simulink model "VSI_LL_IC_"  (R2018a)
settings: Solver=ode23t  StartTime=0  StopTime=0.5  MaxStep=.1e-6  RelTol=1e-4  AbsTol=1e-5  EnableMultiTasking=on
InitFcn:
  | VSI_AFE_parameters_G1_s
values from neighbouring files (symbols this model uses):
  DeadTime = 0.0e-6    (= 0)    [VSI_AFE_parameters_G1_s.m]
  f = 400    [VSI_AFE_parameters_G1_s.m]
  Idref_VSI = 1*11.03    (= 11.03)    [VSI_AFE_parameters_G1_s.m]
  Iqref_VSI = -0    (= 0)    [VSI_AFE_parameters_G1_s.m]
  Ki_PLL_AFE = 1    [VSI_AFE_parameters_G1_s.m]
  Ki_PLL_VSI = 3964    [VSI_AFE_parameters_G1_s.m]
  Kii_AFE = 46.5421*270    (= 12566.367)    [VSI_AFE_parameters_G1_s.m]
  Kii_VSI = 10*628.3185/Vdc    (= 23.2710555556)    [VSI_AFE_parameters_G1_s.m]
  Kipq_VSI = 70    [VSI_AFE_parameters_G1_s.m]
  Kp_PLL_AFE = 0.2    [VSI_AFE_parameters_G1_s.m]
  Kp_PLL_VSI = 8.921    [VSI_AFE_parameters_G1_s.m]
  Kpi_AFE = 0.0116*270    (= 3.132)    [VSI_AFE_parameters_G1_s.m]
  Kpi_VSI = 6.2832/Vdc    (= 0.0232711111111)    [VSI_AFE_parameters_G1_s.m]
  Kppq_VSI = 70*4e-5    (= 0.0028)    [VSI_AFE_parameters_G1_s.m]
  Kpv_AFE = 0.0462    [VSI_AFE_parameters_G1_s.m]
  La = 1000e-6    (= 0.001)    [VSI_AFE_parameters_G1_s.m]
  Lb = 1000e-6    (= 0.001)    [VSI_AFE_parameters_G1_s.m]
  Lc = 1000e-6    (= 0.001)    [VSI_AFE_parameters_G1_s.m]
  PWM_Cycle = 4000    [VSI_AFE_parameters_G1_s.m]
  RLa = 0.100    (= 0.1)    [VSI_AFE_parameters_G1_s.m]
  RLb = 0.100    (= 0.1)    [VSI_AFE_parameters_G1_s.m]
  RLc = 0.100    (= 0.1)    [VSI_AFE_parameters_G1_s.m]
  Vdc = 270/1    (= 270)    [VSI_AFE_parameters_G1_s.m]
  Vfd = 0.75    [VSI_AFE_parameters_G1_s.m]
  Vfs = 1.0    (= 1)    [VSI_AFE_parameters_G1_s.m]
  Vsm = Vse*sqrt(2)-8.2/sqrt(2)*Rss    [VSI_AFE_parameters_G1_s.m]
libraries: powerlib x24, cstblocks x10, simulink x2, powerlib_extras x1
settings Model: Creator=marko  LastModifiedBy=wenbo
settings SolverCC: AutoScaleAbsTol=off  MaxConsecutiveMinStep=10  ZeroCrossAlgorithm=Adaptive  AlgebraicLoopSolver=LineSearch
settings DataIOCC: SaveFinalState=on  SaveFormat=Array  SignalLoggingSaveFormat=ModelDataLogs
settings OptimizationCC: ExpressionDepthLimit=2147483647  LifeSpan=inf
settings DebuggingCC: UnderspecifiedInitializationDetection=Classic  MergeDetectMultiDrivingBlocksExec=none  IgnoredZcDiagnostic=none  SolverPrmCheckMsg=warning  FcnCallInpInsideContextMsg=warning  StateNameClashWarn=warning  SFUnexpectedBacktrackingDiag=warning  SFNoUnconditionalDefaultTransitionDiag=warning  SFExecutionAtInitializationDiag=none
settings HardwareCC: ProdBitPerPointer=32  ProdBitPerSizeT=32  ProdBitPerPtrDiffT=32  ProdLargestAtomicFloat=None  ProdIntDivRoundTo=Undefined  ProdEndianess=Unspecified  ProdWordSize=32  ProdHWDeviceType=32-bit Generic
settings ModelReferenceCC: PropagateSignalLabelsOutOfModel=off
settings CodeAppCC: StateflowObjectComments=on
settings GRTTargetCC: TargetLangStandard=C89/C90 (ANSI)  GeneratePreprocessorConditionals=Disable all  CombineOutputUpdateFcns=off  GRTInterface=on
settings ConfigComp: CovMetricSettings=dw  CovHtmlReporting=on  CovSaveCumulativeToWorkspaceVar=on  CovSaveSingleToWorkspaceVar=on  CovExternalEMLEnable=off
settings SimscapeCC: SimscapeNormalizeSystem=off

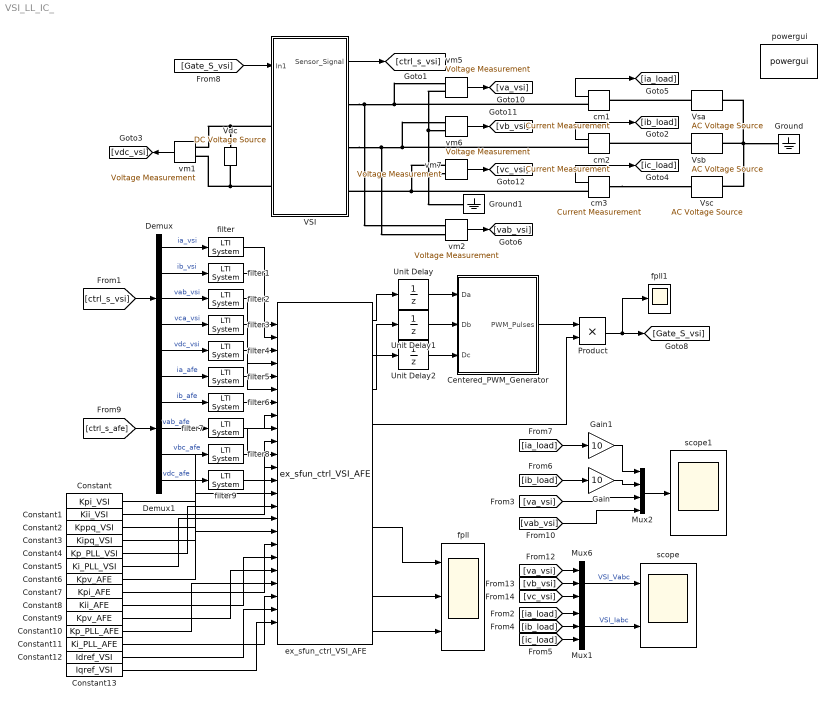
== system VSI_LL_IC_ ==
  Centered_PWM_Generator : Subsystem
  Constant : Constant  Value=Kpi_VSI
  Constant1 : Constant  Value=Kii_VSI
  Constant10 : Constant  Value=Kp_PLL_AFE
  Constant11 : Constant  Value=Ki_PLL_AFE
  Constant12 : Constant  Value=Idref_VSI
  Constant13 : Constant  Value=Iqref_VSI
  Constant2 : Constant  Value=Kppq_VSI
  Constant3 : Constant  Value=Kipq_VSI
  Constant4 : Constant  Value=Kp_PLL_VSI
  Constant5 : Constant  Value=Ki_PLL_VSI
  Constant6 : Constant  Value=Kpv_AFE
  Constant7 : Constant  Value=Kpi_AFE
  Constant8 : Constant  Value=Kii_AFE
  Constant9 : Constant  Value=Kpv_AFE
  Demux : Demux  Outputs=5
  Demux1 : Demux  Outputs=5
  Gain : Gain  Gain=10
  Gain1 : Gain  Gain=10
  Ground : powerlib/Elements/Ground  LConnTagsString=a
  Ground1 : powerlib/Elements/Ground  LConnTagsString=a
  Mux1 : Mux  Inputs=3
  Mux2 : Mux
  Mux6 : Mux  Inputs=3
  Product : Product  RndMeth=Zero
  Unit Delay : UnitDelay  SampleTime=-1
  Unit Delay1 : UnitDelay  SampleTime=-1
  Unit Delay2 : UnitDelay  SampleTime=-1
  VSI : Subsystem
  Vdc : powerlib/Electrical Sources/DC Voltage Source  Amplitude=Vdc  Measurements=None
  Vsa : powerlib/Electrical Sources/AC Voltage Source  Amplitude=Vsm  Phase=90  Frequency=f  SampleTime=0  Measurements=None  BusType=swing  Pref=10e3  Qref=0  Qmin=-inf  Qmax=+inf
  Vsb : powerlib/Electrical Sources/AC Voltage Source  Amplitude=Vsm  Phase=90-120  Frequency=f  SampleTime=0  Measurements=None  BusType=swing  Pref=10e3  Qref=0  Qmin=-inf  Qmax=+inf
  Vsc : powerlib/Electrical Sources/AC Voltage Source  Amplitude=Vsm  Phase=90+120  Frequency=f  SampleTime=0  Measurements=None  BusType=swing  Pref=10e3  Qref=0  Qmin=-inf  Qmax=+inf
  cm1 : powerlib/Measurements/Current Measurement  PhasorSimulation=off  OutputType=Complex  PSBequivalent=0
  cm2 : powerlib/Measurements/Current Measurement  PhasorSimulation=off  OutputType=Complex  PSBequivalent=0
  cm3 : powerlib/Measurements/Current Measurement  PhasorSimulation=off  OutputType=Complex  PSBequivalent=0
  ex_sfun_ctrl_VSI_AFE : S-Function  FunctionName=ex_sfun_ctrl_VSI_AFE  SFunctionDeploymentMode=off  EnableBusSupport=off  mask(Legacy Function){SFunctionSpec=void epwm1_isr(double y1[1], double y2[1], double y3[1], double y4[1], double y5[1], double y6[1], double y7[1], double y8[1], double y9[1], double u1, double u2, double u3, double u4, double u5, double u6, double u7, double u8, double u9, double u10), ShowSpec=off}
      mask prompts: ShowSpec "Display function specification"
      mask help:
      | This block allows you to call the legacy functions specified by the following Legacy Code Tool definition:
      | def.SFunctionName = 'ex_sfun_ctrl_VSI_AFE';
      | def.OutputFcnSpec = 'void epwm1_isr(double y1[1], double y2[1], double y3[1], double y4[1], double y5[1], double y6[1], double y7[1], double y8[1], double y9[1], double u1, double u2, double u3, double u4, double u5, double u6, double u7, double u8, double u9, double u10)';
      | def.HeaderFiles = {'math.h'};
      | def.SourceFiles = {'epwm1_isr.c'};
      | def.SampleTime = 5e-005;
      mask Help: <p>This block was generated automatically by the Legacy Code Tool. For detailed help on this tool, call<a href="matlab:legacy_code('help')"> legacy_code('help')</a>.</p>
      mask Callback ShowSpec:
      | if strcmp(get_param(gcbh, 'ShowSpec'), 'on')
      |   set_param(gcbh, 'MaskDisplay', sprintf('fprintf(''%s'');', get_param(gcbh, 'SFunctionSpec')));
      | else
      |   set_param(gcbh, 'MaskDisplay', sprintf('fprintf(''%s'');', get_param(gcbh, 'FunctionName')));
      | end
      mask Display: fprintf('ex_sfun_ctrl_VSI_AFE');
  filter{,1..9} (10 alike) : cstblocks/LTI System  sys=tf_filter  IC=[]
  fpll : Scope  NumInputPorts=3
  fpll1 : Scope
  powergui : powerlib/powergui  Priority=1  SimulationMode=Continuous  SampleTime=50e-6  frequency=60  Iterations=50  frequencyindice=0  Pbase=100e6  ErrMax=1e-4  UnitsV=kV  UnitsW=MW  buscounter=0  FunctionMessages=off  echomessages=off  EnableUseOfTLC=off  CurrentSourceSwitches=off  DisableSnubberDevices=off  DisableRonSwitches=off  DisableVfSwitches=off  DisplayEquations=off  SolverType=Tustin  Interpol=off  ExternalGateDelay=off  methode=off  Ts=0  x0status=blocks  SPID=on  SwTol=0  HookPort=off  RestoreLinks=warning  ResistiveCurrentMeasurement=off  Frange=[0:2:500]  Ylog=off  Xlog=on  ShowGrid=off  save=off  variable=ZData  structure=ia_L  ZoomFFT=on  StartTime=0.1  cycles=1  DisplayStyle=1  fundamental=400  FreqAxis=off  MaxFrequency=100000  frequencyindicesteady=400  RmsSteady=1  display=off
  scope : Scope  NumInputPorts=2
  scope1 : Scope
  vm{1..2,5..7} (5 alike) : powerlib/Measurements/Voltage Measurement  PhasorSimulation=off  OutputType=Complex  PSBequivalent=0
  wires:
  vm5/1 -> [va_vsi]
  vm6/1 -> [vb_vsi]
  vm7/1 -> [vc_vsi]
  [va_vsi] -> Mux6/1
  [vb_vsi] -> Mux6/2
  [vc_vsi] -> Mux6/3
  Mux6/1 -> scope/1  "VSI_Vabc"
  Unit Delay/1 -> Centered_PWM_Generator/1(Da)
  Unit Delay1/1 -> Centered_PWM_Generator/2(Db)
  Unit Delay2/1 -> Centered_PWM_Generator/3(Dc)
  Demux/1 -> filter/1  "ia_vsi"
  Demux/2 -> filter1/1  "ib_vsi"
  Demux/3 -> filter2/1  "vab_vsi"
  Demux/4 -> filter3/1  "vca_vsi"
  Demux/5 -> filter4/1  "vdc_vsi"
  VSI/1(Sensor_Signal) -> [ctrl_s_vsi]
  [ctrl_s_vsi] -> Demux/1
  [Gate_S_vsi] -> VSI/1(In1)
  Demux1/1 -> filter5/1  "ia_afe"
  Demux1/2 -> filter6/1  "ib_afe"
  Demux1/3 -> filter7/1  "vab_afe"
  Demux1/4 -> filter8/1  "vbc_afe"
  Demux1/5 -> filter9/1  "vdc_afe"
  [ctrl_s_afe] -> Demux1/1
  ex_sfun_ctrl_VSI_AFE/1 -> Unit Delay/1
  ex_sfun_ctrl_VSI_AFE/2 -> Unit Delay1/1
  ex_sfun_ctrl_VSI_AFE/3 -> Unit Delay2/1
  filter/1 -> ex_sfun_ctrl_VSI_AFE/1
  filter1/1 -> ex_sfun_ctrl_VSI_AFE/2
  filter2/1 -> ex_sfun_ctrl_VSI_AFE/3
  filter3/1 -> ex_sfun_ctrl_VSI_AFE/4
  filter4/1 -> ex_sfun_ctrl_VSI_AFE/5
  filter5/1 -> ex_sfun_ctrl_VSI_AFE/6
  filter6/1 -> ex_sfun_ctrl_VSI_AFE/7
  filter7/1 -> ex_sfun_ctrl_VSI_AFE/8
  filter8/1 -> ex_sfun_ctrl_VSI_AFE/9
  filter9/1 -> ex_sfun_ctrl_VSI_AFE/10
  vm1/1 -> [vdc_vsi]
  Mux1/1 -> scope/2  "VSI_Iabc"
  [ia_load] -> Mux1/1
  [ib_load] -> Mux1/2
  [ic_load] -> Mux1/3
  Product/1 -> [Gate_S_vsi], fpll1/1
  Centered_PWM_Generator/1(PWM_Pulses) -> Product/1
  ex_sfun_ctrl_VSI_AFE/4 -> Product/2
  Constant/1 -> ex_sfun_ctrl_VSI_AFE/11
  Constant1/1 -> ex_sfun_ctrl_VSI_AFE/12
  Constant2/1 -> ex_sfun_ctrl_VSI_AFE/13
  Constant3/1 -> ex_sfun_ctrl_VSI_AFE/14
  Constant4/1 -> ex_sfun_ctrl_VSI_AFE/15
  Constant5/1 -> ex_sfun_ctrl_VSI_AFE/16
  Constant6/1 -> ex_sfun_ctrl_VSI_AFE/17
  Constant7/1 -> ex_sfun_ctrl_VSI_AFE/18
  Constant8/1 -> ex_sfun_ctrl_VSI_AFE/19
  Constant9/1 -> ex_sfun_ctrl_VSI_AFE/20
  Constant10/1 -> ex_sfun_ctrl_VSI_AFE/21
  Constant11/1 -> ex_sfun_ctrl_VSI_AFE/22
  Constant12/1 -> ex_sfun_ctrl_VSI_AFE/23
  Constant13/1 -> ex_sfun_ctrl_VSI_AFE/24
  [ib_load] -> Gain/1
  Mux2/1 -> scope1/1
  ex_sfun_ctrl_VSI_AFE/9 -> fpll/2
  ex_sfun_ctrl_VSI_AFE/10 -> fpll/3
  ex_sfun_ctrl_VSI_AFE/7 -> fpll/1
  vm2/1 -> [vab_vsi]
  [ia_load] -> Gain1/1
  Gain1/1 -> Mux2/1
  Gain/1 -> Mux2/2
  [va_vsi] -> Mux2/3
  [vab_vsi] -> Mux2/4
  cm1/1 -> [ia_load]
  cm2/1 -> [ib_load]
  cm3/1 -> [ic_load]
  connections:
  VSI/LConn1 -- Vdc/RConn1 -- vm1/LConn1
  VSI/LConn2 -- Vdc/LConn1 -- vm1/LConn2
  vm7/LConn1 -- cm3/RConn1 -- VSI/RConn3
  VSI/RConn2 -- vm2/LConn2 -- vm6/LConn1 -- cm2/RConn1
  VSI/RConn1 -- vm2/LConn1 -- vm5/LConn1 -- cm1/RConn1
  Vsa/LConn1 -- Vsc/LConn1 -- Vsb/LConn1 -- Ground/LConn1
  vm5/LConn2 -- vm6/LConn2 -- Ground1/LConn1 -- vm7/LConn2
  cm3/LConn1 -- Vsc/RConn1
  Vsb/RConn1 -- cm2/LConn1
  Vsa/RConn1 -- cm1/LConn1

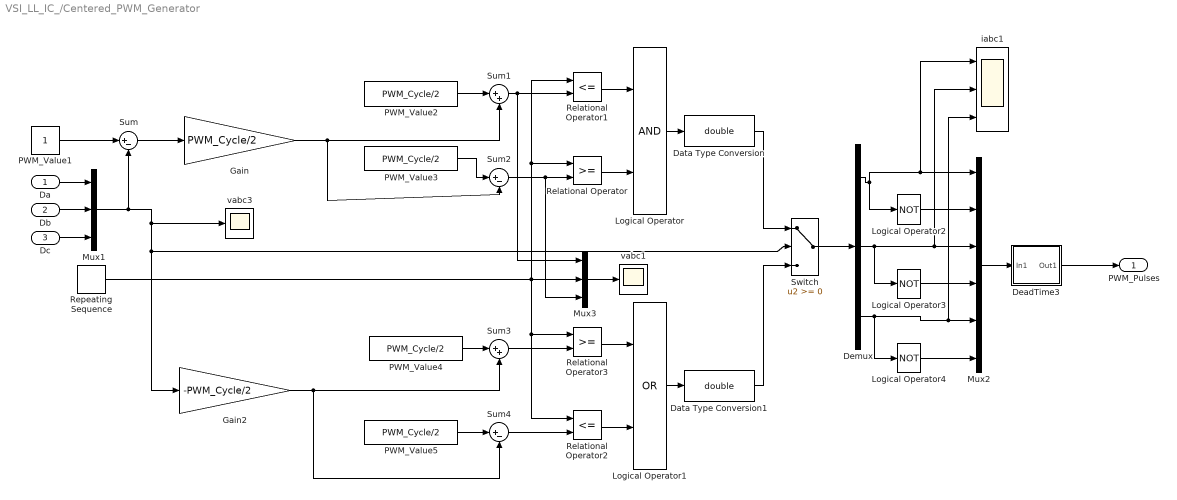
== system VSI_LL_IC_/Centered_PWM_Generator ==
  Da : Inport
  Db : Inport  Port=2
  Dc : Inport  Port=3
  Data Type Conversion : DataTypeConversion  OutDataTypeStr=double
  Data Type Conversion1 : DataTypeConversion  OutDataTypeStr=double
  DeadTime3 : Subsystem
  Demux : Demux  Outputs=3
  Gain : Gain  Gain=PWM_Cycle/2
  Gain2 : Gain  Gain=-PWM_Cycle/2
  Logical Operator : Logic  AllPortsSameDT=off  OutDataTypeStr=boolean
  Logical Operator1 : Logic  Operator=OR  AllPortsSameDT=off  OutDataTypeStr=boolean
  Logical Operator2 : Logic  Operator=NOT  OutDataTypeStr=float('double')
  Logical Operator3 : Logic  Operator=NOT  OutDataTypeStr=float('double')
  Logical Operator4 : Logic  Operator=NOT  OutDataTypeStr=float('double')
  Mux1 : Mux  Inputs=3
  Mux2 : Mux  Inputs=6
  Mux3 : Mux  Inputs=3
  PWM_Value1 : Constant
  PWM_Value{2..5} (4 alike) : Constant  Value=PWM_Cycle/2
  Relational Operator : RelationalOperator  OutDataTypeStr=boolean  RndMeth=Nearest
  Relational Operator1 : RelationalOperator  Operator=<=  OutDataTypeStr=boolean  RndMeth=Nearest
  Relational Operator2 : RelationalOperator  Operator=<=  OutDataTypeStr=boolean  RndMeth=Nearest
  Relational Operator3 : RelationalOperator  OutDataTypeStr=boolean  RndMeth=Nearest
  Repeating Sequence : simulink/Sources/Repeating Sequence  rep_seq_t="[0  (0.5*PWM_Cycle*12.5e-9) (1*PWM_Cycle*12.5e-9)]"  rep_seq_y=[0 PWM_Cycle 0]
  Sum : Sum  Inputs=|+-
  Sum1 : Sum  Inputs=|++
  Sum2 : Sum  Inputs=|+-
  Sum3 : Sum  Inputs=|++
  Sum4 : Sum  Inputs=|+-
  Switch : Switch
  iabc1 : Scope  NumInputPorts=3
  vabc1 : Scope
  vabc3 : Scope
  PWM_Pulses : Outport
  wires:
  Logical Operator4/1 -> Mux2/6
  Demux/3 -> Logical Operator4/1, Mux2/5, iabc1/3
  Logical Operator3/1 -> Mux2/4
  Demux/2 -> Logical Operator3/1, Mux2/3, iabc1/2
  Logical Operator2/1 -> Mux2/2
  Demux/1 -> Logical Operator2/1, Mux2/1, iabc1/1
  Mux2/1 -> DeadTime3/1(In1)
  Dc/1 -> Mux1/3
  Db/1 -> Mux1/2
  Da/1 -> Mux1/1
  Mux1/1 -> Sum/2, Switch/2, Gain2/1, vabc3/1
  Switch/1 -> Demux/1
  Data Type Conversion1/1 -> Switch/3
  Gain2/1 -> Sum3/2, Sum4/2
  Logical Operator1/1 -> Data Type Conversion1/1
  Relational Operator2/1 -> Logical Operator1/2
  Relational Operator3/1 -> Logical Operator1/1
  Sum3/1 -> Relational Operator3/2
  Sum4/1 -> Relational Operator2/2
  PWM_Value5/1 -> Sum4/1
  PWM_Value4/1 -> Sum3/1
  Data Type Conversion/1 -> Switch/1
  Logical Operator/1 -> Data Type Conversion/1
  Relational Operator/1 -> Logical Operator/2
  Relational Operator1/1 -> Logical Operator/1
  Sum1/1 -> Relational Operator1/2, Mux3/1
  Sum2/1 -> Relational Operator/2, Mux3/3
  PWM_Value3/1 -> Sum2/1
  Gain/1 -> Sum2/2, Sum1/2
  Sum/1 -> Gain/1
  PWM_Value1/1 -> Sum/1
  Repeating Sequence/1 -> Relational Operator1/1, Relational Operator/1, Relational Operator3/1, Relational Operator2/1, Mux3/2
  DeadTime3/1(Out1) -> PWM_Pulses/1
  PWM_Value2/1 -> Sum1/1
  Mux3/1 -> vabc1/1

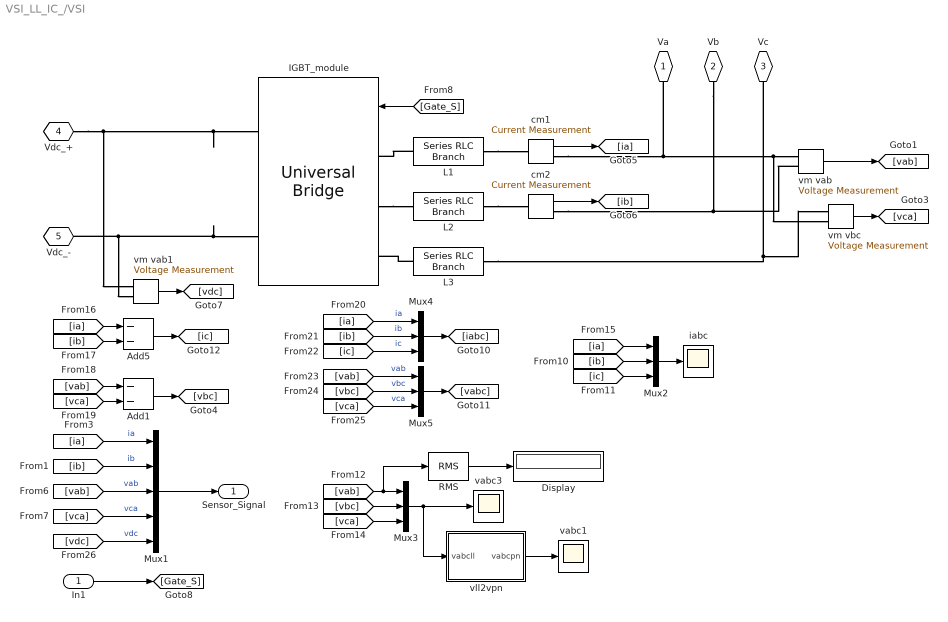
== system VSI_LL_IC_/VSI ==
  In1 : Inport
  Add1 : Sum  Inputs=--
  Add5 : Sum  Inputs=--
  Display : Display
  IGBT_module : powerlib/Power Electronics/Universal Bridge  Arms=3  SnubberResistance=inf  SnubberCapacitance=inf  Device=IGBT / Diodes  Ron=Rsd  Lon=0  ForwardVoltages=[Vfs Vfd]  ForwardVoltage=0  GTOparameters=[ 10e-6 , 20e-6 ]  IGBTparameters=[ 0, 0 ]  Measurements=None  Measurements_2=None  converterType=Rectifier
  L1 : powerlib/Elements/Series RLC Branch  LConnTagsString=__new0  RConnTagsString=__new0  BranchType=RL  Resistance=RLa  Inductance=La  SetiL0=off  InitialCurrent=0  Capacitance=1e-6  Setx0=off  InitialVoltage=0  Measurements=None
  L2 : powerlib/Elements/Series RLC Branch  LConnTagsString=__new0  RConnTagsString=__new0  BranchType=RL  Resistance=RLb  Inductance=Lb  SetiL0=off  InitialCurrent=0  Capacitance=1e-6  Setx0=off  InitialVoltage=0  Measurements=None
  L3 : powerlib/Elements/Series RLC Branch  LConnTagsString=__new0  RConnTagsString=__new0  BranchType=RL  Resistance=RLc  Inductance=Lc  SetiL0=off  InitialCurrent=0  Capacitance=1e-6  Setx0=off  InitialVoltage=0  Measurements=None
  Mux1 : Mux  Inputs=5
  Mux{2..5} (4 alike) : Mux  Inputs=3
  RMS : powerlib_extras/Measurements/RMS  f1=60
  cm1 : powerlib/Measurements/Current Measurement  PhasorSimulation=off  OutputType=Complex  PSBequivalent=0
  cm2 : powerlib/Measurements/Current Measurement  PhasorSimulation=off  OutputType=Complex  PSBequivalent=0
  iabc : Scope
  vabc1 : Scope
  vabc3 : Scope
  vll2vpn : Subsystem
  vm vab : powerlib/Measurements/Voltage Measurement  PhasorSimulation=off  OutputType=Complex  PSBequivalent=0
  vm vab1 : powerlib/Measurements/Voltage Measurement  PhasorSimulation=off  OutputType=Complex  PSBequivalent=0
  vm vbc : powerlib/Measurements/Voltage Measurement  PhasorSimulation=off  OutputType=Complex  PSBequivalent=0
  Va : PMIOPort  Tag=PMCPort  Side=Right
  Vb : PMIOPort  Tag=PMCPort  Port=2  Side=Right
  Vc : PMIOPort  Tag=PMCPort  Port=3  Side=Right
  Vdc_+ : PMIOPort  Tag=PMCPort  Port=4  Side=Left
  Vdc_- : PMIOPort  Tag=PMCPort  Port=5  Side=Left
  Sensor_Signal : Outport
  wires:
  cm1/1 -> [ia]
  [Gate_S] -> IGBT_module/1
  Mux2/1 -> iabc/1
  Mux3/1 -> vabc3/1, vll2vpn/1(vabcll)
  [ia] -> Mux2/1
  [ib] -> Mux2/2
  [ic] -> Mux2/3
  [vab] -> Mux3/1, RMS/1
  [vbc] -> Mux3/2
  [vca] -> Mux3/3
  [ia] -> Mux4/1  "ia"
  [ib] -> Mux4/2  "ib"
  [ic] -> Mux4/3  "ic"
  Mux4/1 -> [iabc]
  [vab] -> Mux5/1  "vab"
  [vbc] -> Mux5/2  "vbc"
  [vca] -> Mux5/3  "vca"
  Mux5/1 -> [vabc]
  vll2vpn/1(vabcpn) -> vabc1/1
  RMS/1 -> Display/1
  cm2/1 -> [ib]
  vm vab/1 -> [vab]
  vm vbc/1 -> [vca]
  vm vab1/1 -> [vdc]
  [ia] -> Mux1/1  "ia"
  [ib] -> Mux1/2  "ib"
  [vab] -> Mux1/3  "vab"
  [vca] -> Mux1/4  "vca"
  [vdc] -> Mux1/5  "vdc"
  Mux1/1 -> Sensor_Signal/1
  In1/1 -> [Gate_S]
  Add5/1 -> [ic]
  [ia] -> Add5/1
  [ib] -> Add5/2
  Add1/1 -> [vbc]
  [vab] -> Add1/1
  [vca] -> Add1/2
  connections:
  Va/RConn1 -- cm1/RConn1 -- vm vab/LConn1 -- vm vbc/LConn2
  vm vab/LConn2 -- Vb/RConn1 -- cm2/RConn1
  L1/LConn1 -- IGBT_module/LConn1
  L1/RConn1 -- cm1/LConn1
  L2/RConn1 -- cm2/LConn1
  IGBT_module/LConn2 -- L2/LConn1
  L3/LConn1 -- IGBT_module/LConn3
  Vdc_+/RConn1 -- IGBT_module/RConn1 -- vm vab1/LConn1
  IGBT_module/RConn2 -- Vdc_-/RConn1 -- vm vab1/LConn2
  Vc/RConn1 -- L3/RConn1 -- vm vbc/LConn1

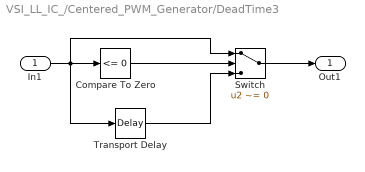
== system VSI_LL_IC_/Centered_PWM_Generator/DeadTime3 ==
  In1 : Inport
  Compare To Zero : simulink/Logic and Bit Operations/Compare To Zero  relop=<=  OutDataTypeStr=uint8
  Switch : Switch  Criteria=u2 ~= 0
  Transport Delay : TransportDelay  DelayTime=DeadTime  BufferSize=2048*16  FixedBuffer=on
  Out1 : Outport
  wires:
  Switch/1 -> Out1/1
  Compare To Zero/1 -> Switch/2
  Transport Delay/1 -> Switch/3
  In1/1 -> Transport Delay/1, Compare To Zero/1, Switch/1

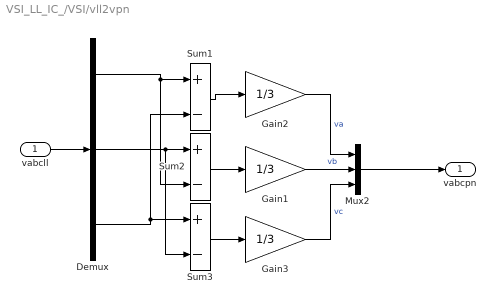
== system VSI_LL_IC_/VSI/vll2vpn ==
  vabcll : Inport
  Demux : Demux  Outputs=3
  Gain1 : Gain  Gain=1/3
  Gain2 : Gain  Gain=1/3
  Gain3 : Gain  Gain=1/3
  Mux2 : Mux  Inputs=3
  Sum1 : Sum  Inputs=+-
  Sum2 : Sum  Inputs=+-
  Sum3 : Sum  Inputs=+-
  vabcpn : Outport
  wires:
  Mux2/1 -> vabcpn/1
  vabcll/1 -> Demux/1
  Demux/1 -> Sum1/1, Sum2/2
  Demux/3 -> Sum1/2, Sum3/1
  Sum1/1 -> Gain2/1
  Demux/2 -> Sum2/1, Sum3/2
  Sum2/1 -> Gain1/1
  Sum3/1 -> Gain3/1
  Gain2/1 -> Mux2/1  "va"
  Gain1/1 -> Mux2/2  "vb"
  Gain3/1 -> Mux2/3  "vc"
